simulink model "frdm_receive_data"  (R2017a)
settings: Solver=VariableStepAuto  StartTime=0.0  StopTime=inf  RelTol=1e-3
libraries: frdmkl25zlib x1
settings Model: SimulationMode=external  Creator=WARA  LastModifiedBy=WARA

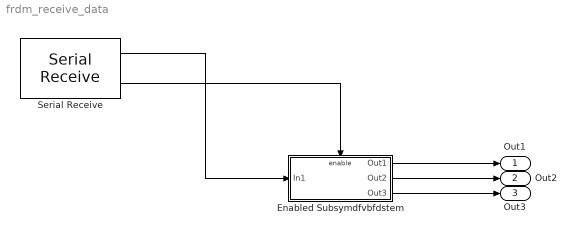
== system frdm_receive_data ==
  Enabled Subsymdfvbfdstem : Subsystem  TreatAsAtomicUnit=on
  Serial Receive : frdmkl25zlib/Serial Receive  uart=UART2  DataType=int8  DataLength=3  SampleTime=0.1
      settings: SourceProductName=Simulink Coder Support Package for NXP FRDM-KL25Z Board  SourceProductBaseCode=EC_FREEDOM_BOARD
  Out1 : Outport
  Out2 : Outport  Port=2
  Out3 : Outport  Port=3
  wires:
  Serial Receive/1 -> Enabled Subsymdfvbfdstem/1(In1)
  Serial Receive/2 -> Enabled Subsymdfvbfdstem/Enable
  Enabled Subsymdfvbfdstem/1(Out1) -> Out1/1
  Enabled Subsymdfvbfdstem/2(Out2) -> Out2/1
  Enabled Subsymdfvbfdstem/3(Out3) -> Out3/1

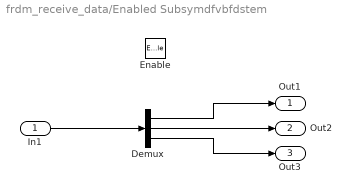
== system frdm_receive_data/Enabled Subsymdfvbfdstem ==
  In1 : Inport
  Enable : EnablePort
  Demux : Demux  Outputs=3
  Out1 : Outport
  Out2 : Outport  Port=2
  Out3 : Outport  Port=3
  wires:
  In1/1 -> Demux/1
  Demux/1 -> Out1/1
  Demux/2 -> Out2/1
  Demux/3 -> Out3/1
